simulink model "teamduoMV"  (R2024b)
settings: Solver=VariableStepAuto  StartTime=0.0  StopTime=60  RelTol=1e-3
settings Model: Creator=sprinkle  LastModifiedBy=jasonmok
settings OptimizationCC: ReuseModelBlockBuffer=off
settings RTWCC: GPUComputeCapability=3.5

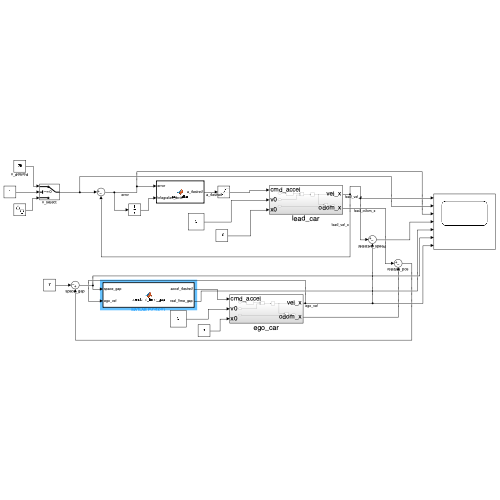
[thumbnail: Simulink's stored preview of the top-level diagram]
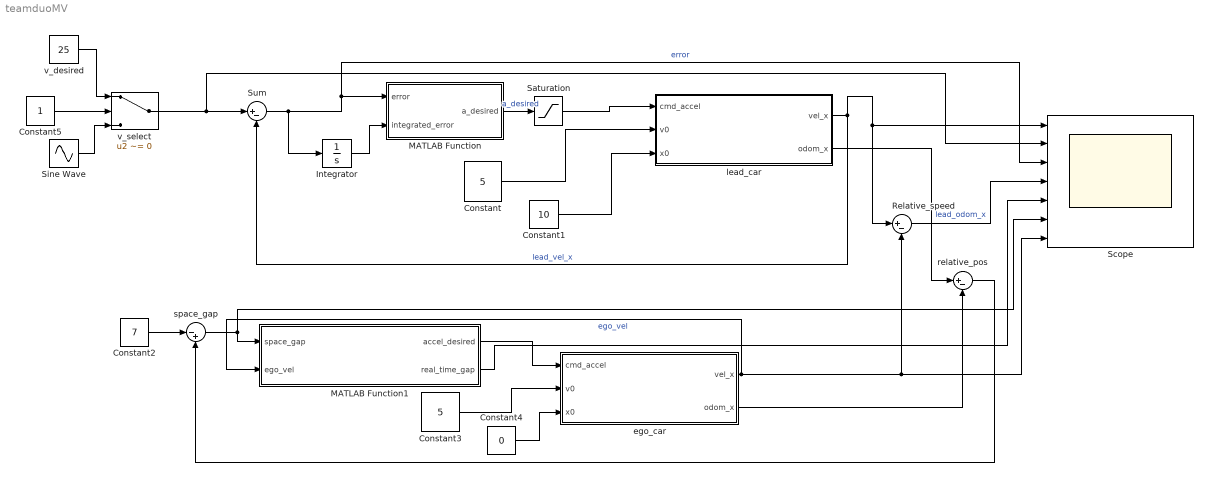
== system teamduoMV ==
  Constant : Constant  Value=5
  Constant1 : Constant  Value=10
  Constant2 : Constant  Value=7
  Constant3 : Constant  Value=5
  Constant4 : Constant  Value=0
  Constant5 : Constant
  Integrator : Integrator
  MATLAB Function : MATLAB Function  TreatAsAtomicUnit=on
  MATLAB Function1 : MATLAB Function  TreatAsAtomicUnit=on
  Relative_speed : Sum  Inputs=|+-
  Saturation : Saturate  UpperLimit=1.5  LowerLimit=-3
  Scope : Scope  NumInputPorts=7
  Sine Wave : Sin  Bias=20  SampleTime=0
  Sum : Sum  Inputs=|+-
  ego_car : Subsystem
  lead_car : Subsystem
  relative_pos : Sum  Inputs=|+-
  space_gap : Sum  Inputs=|-+
  v_desired : Constant  Value=25
  v_select : Switch  Criteria=u2 ~= 0  Threshold=0.5  SaturateOnIntegerOverflow=off  InputSameDT=off
  wires:
  Constant/1 -> lead_car/2(v0)
  Constant1/1 -> lead_car/3(x0)
  lead_car/1(vel_x) -> Relative_speed/1, Scope/1, Sum/2  "lead_vel_x"
  lead_car/2(odom_x) -> relative_pos/1  "lead_odom_x"
  v_select/1 -> Scope/2, Sum/1
  Sum/1 -> Integrator/1, Scope/3, MATLAB Function/1(error)  "error"
  Integrator/1 -> MATLAB Function/2(integrated_error)
  ego_car/1(vel_x) -> MATLAB Function1/2(ego_vel), Scope/7, Relative_speed/2  "ego_vel"
  ego_car/2(odom_x) -> relative_pos/2
  Constant2/1 -> space_gap/1
  relative_pos/1 -> space_gap/2
  space_gap/1 -> Scope/6, MATLAB Function1/1(space_gap)
  MATLAB Function1/1(accel_desired) -> ego_car/1(cmd_accel)
  Constant3/1 -> ego_car/2(v0)
  Constant4/1 -> ego_car/3(x0)
  Relative_speed/1 -> Scope/4
  Constant5/1 -> v_select/2
  Sine Wave/1 -> v_select/3
  v_desired/1 -> v_select/1
  MATLAB Function/1(a_desired) -> Saturation/1  "a_desired"
  Saturation/1 -> lead_car/1(cmd_accel)
  MATLAB Function1/2(real_time_gap) -> Scope/5

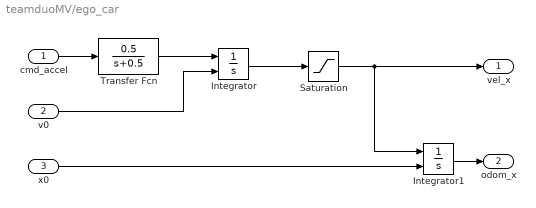
== system teamduoMV/ego_car ==
  cmd_accel : Inport
  v0 : Inport  Port=2
  x0 : Inport  Port=3
  Integrator : Integrator  InitialConditionSource=external
  Integrator1 : Integrator  InitialConditionSource=external
  Saturation : Saturate  UpperLimit=80  LowerLimit=0
  Transfer Fcn : TransferFcn  Numerator=[0.5]  Denominator=[1 0.5]
  vel_x : Outport
  odom_x : Outport  Port=2
  wires:
  v0/1 -> Integrator/2
  cmd_accel/1 -> Transfer Fcn/1
  Transfer Fcn/1 -> Integrator/1
  Integrator1/1 -> odom_x/1
  Integrator/1 -> Saturation/1
  x0/1 -> Integrator1/2
  Saturation/1 -> vel_x/1, Integrator1/1

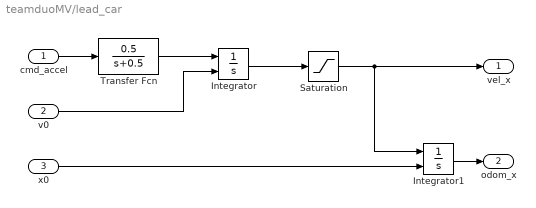
== system teamduoMV/lead_car ==
  cmd_accel : Inport
  v0 : Inport  Port=2
  x0 : Inport  Port=3
  Integrator : Integrator  InitialConditionSource=external
  Integrator1 : Integrator  InitialConditionSource=external
  Saturation : Saturate  UpperLimit=80  LowerLimit=0
  Transfer Fcn : TransferFcn  Numerator=[0.5]  Denominator=[1 0.5]
  vel_x : Outport
  odom_x : Outport  Port=2
  wires:
  v0/1 -> Integrator/2
  cmd_accel/1 -> Transfer Fcn/1
  Transfer Fcn/1 -> Integrator/1
  Integrator1/1 -> odom_x/1
  Integrator/1 -> Saturation/1
  x0/1 -> Integrator1/2
  Saturation/1 -> vel_x/1, Integrator1/1

== matlab function teamduoMV/MATLAB Function ==
  data: error input; a_desired output; integrated_error input
function a_desired = controller(error,integrated_error)

a_desired = 0.3*error + 0.01*integrated_error;

== matlab function teamduoMV/MATLAB Function1 ==
  data: space_gap input; accel_desired output; real_time_gap output; ego_vel input
function [accel_desired, real_time_gap] = constant_time_gap(space_gap, ego_vel)

tau=2;
alpha=4;

real_time_gap = space_gap/ego_vel;
error = real_time_gap - tau;
accel_desired = alpha*(error);
